simulink model "nms3D_2021"  (R2021a)
settings: Solver=ode15s  StartTime=0.0  StopTime=2  MaxStep=1e-2  RelTol=1e-2
StartFcn:
  | tic
StopFcn:
  | toc
  | 
  | 
  | %if GimbalLockFlag
  |  % fprintf(2, 'Almost reached Gimbal Lock of IMU. Simulation stopped.\n')
  | %end
  | 
  | %fprintf('Elapsed time: %4.2f sec (%4.2f%% realtime)\n', a, tout(end)/a*100)
values from neighbouring files (symbols this model uses):
  Balance02 = pMod(24:29)    [AssignSimulinkParams.m]    (also in assign_parameters.m = param(26:29))
  Balance13 = pMod(30:35)    [AssignSimulinkParams.m]    (also in assign_parameters.m = param(30:33))
  BalanceTrunk = pMod(22:23)    [AssignSimulinkParams.m]    (also in assign_parameters.m = param(22:23))
  BalanceTrunkLat = param(24:25)    [assign_parameters.m]
  BalanceTrunkLatOld = pMod(43:46)    [AssignSimulinkParams.m]    (also in assign_parameters.m = param(43:46))
  BalanceTrunkOld = param(49:53)    [assign_parameters.m]
  BasisStim = pMod(1:11)    [AssignSimulinkParams.m]    (also in assign_parameters.m = param(1:11))
  CompliantLeg = pMod(12:14)    [AssignSimulinkParams.m]    (also in assign_parameters.m = param(12:14))
  CompliantLegLat = pMod(15)    [AssignSimulinkParams.m]    (also in assign_parameters.m = param(15))
  PreventKneeOverextension = pMod(16:21)    [AssignSimulinkParams.m]    (also in assign_parameters.m = param(16:21))
  SwingCompLatOld = param(47:48)    [assign_parameters.m]
  Target02 = pMod(36:38)    [AssignSimulinkParams.m]    (also in assign_parameters.m = param(34:36))
  Target02_va = pMod(49:54)    [AssignSimulinkParams.m]    (also in assign_parameters.m = param(60:65))
  Target13 = pMod(39:41)    [AssignSimulinkParams.m]    (also in assign_parameters.m = param(37:39))
  Target13_va = pMod(55:60)    [AssignSimulinkParams.m]    (also in assign_parameters.m = param(66:71))
  theta0_world = param(59)    [assign_parameters.m]
  WramameiSL_1000 = readmatrix('WSL_1000_Norm_Sigmoid_MSE_cont.csv')    [nms3D_prep.m]
  ZramameiSL_1000 = readmatrix('ZSL_1000_Norm_Sigmoid_MSE_cont.csv')    [nms3D_prep.m]
undefined symbols (not defined in the file or in its folder): ICs, mParams, X, Y, Z
libraries: nesl_utility x106, sm_lib x87, simulink x70, eeGeneralControl x28, robotmaniplib x14, dspinverses x10, robotcorelib x5, dspmathops x3, vrlib x1, pid_lib x1
(part 7 of 8)

== system nms3D_2021/Supraspinal Level/Subsystem/Stance Leg Control/PD-Controller For Saggital Trunk Balance ==
  Gain : Gain  Gain=-1
  Low-Pass Filter (Discrete or Continuous) : eeGeneralControl/Low-Pass Filter (Discrete or Continuous)  K=1  T=0.01  B=inf  A=-inf  init_option=Inherited from block input  x0=0  Ts=-1
  Minus : Sum  Inputs=+-
  PID Controller : pid_lib/PID Controller  Controller=PD  Form=Parallel  TimeDomain=Continuous-time  UseExternalTs=off  SampleTime=-1  IntegratorMethod=Forward Euler  FilterMethod=Forward Euler  ControllerParametersSource=internal  P=40  I=0  D=80  UseFilter=on  N=100  TunerSelectOption=Transfer Function Based (PID Tuner App)  ZeroCross=off  InitialConditionSource=internal  InitialConditionForIntegrator=0  InitialConditionForFilter=0  DifferentiatorICPrevScaledInput=0  ExternalReset=none  TrackingMode=off  Kt=1  LimitOutput=off  SatLimitsSource=internal  UpperSaturationLimit=inf  LowerSaturationLimit=-inf  LinearizeAsGain=on  AntiWindupMode=none  Kb=1  POutMin=[]  POutMax=[]  IOutMin=[]  IOutMax=[]  DOutMin=[]  DOutMax=[]  NOutMin=[]  NOutMax=[]  SumOutMin=[]  SumOutMax=[]  SaturationOutMin=[]  SaturationOutMax=[]  PParamMin=[]  PParamMax=[]  IParamMin=[]  IParamMax=[]  DParamMin=[]  DParamMax=[]  NParamMin=[]  NParamMax=[]  KbParamMin=[]  KbParamMax=[]  KtParamMin=[]  KtParamMax=[]  KbOutMin=[]  KbOutMax=[]  KtOutMin=[]  KtOutMax=[]  IntegratorOutMin=[]  IntegratorOutMax=[]  FilterOutMin=[]  FilterOutMax=[]  SumI1OutMin=[]  SumI1OutMax=[]  SumI2OutMin=[]  SumI2OutMax=[]  SumI3OutMin=[]  SumI3OutMax=[]  SumI4OutMin=[]  SumI4OutMax=[]  SumDOutMin=[]  SumDOutMax=[]  DifferentiatorOutMin=[]  DifferentiatorOutMax=[]  FilterDiffOutCoefMin=[]  FilterDiffOutCoefMax=[]  ReciprocalOutMin=[]  ReciprocalOutMax=[]  SumDenOutMin=[]  SumDenOutMax=[]  SumNumOutMin=[]  SumNumOutMax=[]  DivideOutMin=[]  DivideOutMax=[]  UdiffTsProdOutMin=[]  UdiffTsProdOutMax=[]  NTsProdOutMin=[]  NTsProdOutMax=[]  UintegralTsProdOutMin=[]  UintegralTsProdOutMax=[]  UngainTsProdOutMin=[]  UngainTsProdOutMax=[]  IntegratorContinuousStateAttributes=''  IntegratorStateMustResolveToSignalObject=off  IntegratorRTWStateStorageClass=Auto  FilterContinuousStateAttributes=''  FilterStateMustResolveToSignalObject=off  FilterRTWStateStorageClass=Auto  ParallelPVariant=InternalParameters  IdealPVariant=Disabled  IVariant=Disabled  DVariant=InternalParameters  IntegratorVariant=Disabled  SatVariant=Disabled  AWVariant=Disabled  PCopyVariant=Disabled  TRVariant=Disabled  FdbkBlocksVariant=Forward  IdealPFdbkVariant=Disabled  SatFdbkVariant=Disabled  DerivativeFilterVariant=ContFilter  NVariant=InternalParameters  NCopyVariant=Disabled  FilterICVariant=InternalICsFilter  IntegratorICVariant=Disabled  ExternalResetVariant=Disabled  TRSumVariant=Passthrough  SumFdbkVariant=Disabled  SumVariant=Sum_PD  TsampFilterVariant=InternalTs  TsampNgainVariant=Passthrough  TsampIntegralVariant=Disabled_SignalSpec  ExternalSaturationOutDataTypeStr=Inherit: Same as second input
  Scope{,1..3} (4 alike) : Scope
  To Workspace6 : ToWorkspace  VariableName=RotSag  SampleTime=-1
      settings: Save2DSignal=2-D array (concatenate along first dimension)
  PD Input : Outport
  wires:
  Gain/1 -> Low-Pass Filter (Discrete or Continuous)/1
  Minus/1 -> Scope2/1, PID Controller/1
  [TrunkRot_sag] -> To Workspace6/1, Minus/1, Scope/1
  PID Controller/1 -> Scope3/1, Gain/1
  [theta0_world] -> Scope1/1, Minus/2
  Low-Pass Filter (Discrete or Continuous)/1 -> PD Input/1

== system nms3D_2021/Supraspinal Level/Subsystem/Stance Leg Control/Stance Leg ==
  left/right : Inport
  Balance Control [Ankle Strategy] : Inport  Port=2
  PD Input : Inport  Port=3
  Foot Orientation Left : Subsystem
  Foot Orientation Right : Subsystem
  Inverse Dynamics Left Leg : Subsystem
  Mux : Mux  Inputs=2
  Mux1 : Mux  Inputs=2
  NOT : Logic  Operator=NOT  AllPortsSameDT=off  OutDataTypeStr=boolean
  NOT2 : Logic  Operator=NOT  AllPortsSameDT=off  OutDataTypeStr=boolean
  Selector : Selector  InputPortWidth=5  IndexOptions=Index vector (dialog)  Indices=[5 4 3 2 1]  OutputSizes=1
  Selector1 : Selector  InputPortWidth=5  IndexOptions=Index vector (dialog)  Indices=[5 4 3 2 1]  OutputSizes=1
  Subsystem : Subsystem
  Transpose : Math  Operator=transpose  SaturateOnIntegerOverflow=on
  long delay 1 : eeGeneralControl/Low-Pass Filter (Discrete or Continuous)  K=1  T=mParams.control.delays.long  B=inf  A=-inf  init_option=Inherited from block input  x0=0  Ts=0
  long delay 2 : eeGeneralControl/Low-Pass Filter (Discrete or Continuous)  K=1  T=mParams.control.delays.long  B=inf  A=-inf  init_option=Inherited from block input  x0=0  Ts=0
  long delay 4 : eeGeneralControl/Low-Pass Filter (Discrete or Continuous)  K=1  T=mParams.control.delays.long  B=inf  A=-inf  init_option=Inherited from block input  x0=0  Ts=0
  Stance Torques Left : Outport
  Stance Torques Right : Outport  Port=2
  wires:
  Selector/1 -> Mux/2
  Selector1/1 -> Mux1/2
  [R_body] -> long delay 4/1
  left/right/1 -> NOT/1, NOT2/1, Inverse Dynamics Left Leg/2(left/right)
  Transpose/1 -> Foot Orientation Right/1(R Pelvis), Foot Orientation Left/1(R Pelvis)
  Foot Orientation Left/1(Orientation Foot (Z)) -> Mux1/1
  Foot Orientation Right/1(Foot Orientation (Z)) -> Mux/1
  Balance Control [Ankle Strategy]/1 -> Inverse Dynamics Left Leg/3(Task), Subsystem/4(Task)
  Inverse Dynamics Left Leg/1(Stance Torques Left) -> Stance Torques Left/1
  Mux/1 -> Subsystem/1(Config [5])
  NOT2/1 -> Subsystem/3(left/right)
  Subsystem/1(Stance Torques Right) -> Stance Torques Right/1
  Mux1/1 -> Inverse Dynamics Left Leg/1(Config [5])
  long delay 1/1 -> Selector1/1
  long delay 2/1 -> Selector/1
  long delay 4/1 -> Transpose/1
  [Llegq] -> long delay 1/1
  [Rlegq] -> long delay 2/1
  PD Input/1 -> Subsystem/2(PD Input), Inverse Dynamics Left Leg/4(PD Input)

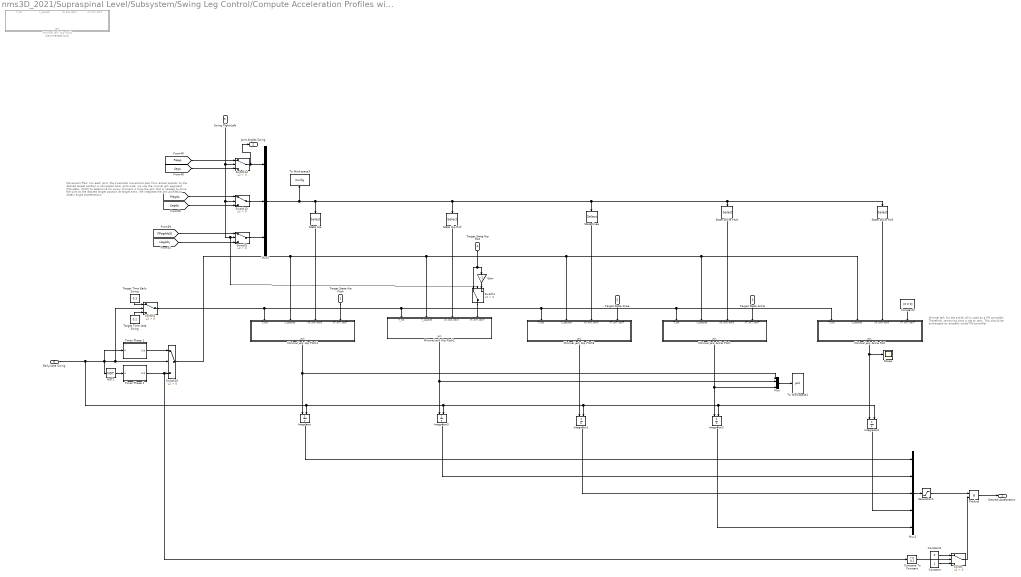
== system nms3D_2021/Supraspinal Level/Subsystem/Swing Leg Control/Compute Acceleration Profiles with Minimal Jerk Approach ==
  note: Movement Plan: For each joint, the kinematic movement plan from actual position to the desired target position is computed here. Joint-wise, we use the mininal jerk approach [Movellan, 2012] to determine for every moment in time the jerk that is needed to drive the joint to the desired target position at target time. We integrate the jerk profiles to obtain angle accelerations.
  note: Minimal Jerk for the ankle roll is used as a PD controller. Therefore, remaining time is set to zero. This should be exchanged by properly tuned PD-controller
  Target State Hip Pitch : Inport
  Target State Knee : Inport  Port=2
  Target State Ankle : Inport  Port=3
  Target State Hip Roll : Inport  Port=4
  Swing Right/Left : Inport  Port=5
  Early/Late Swing : Inport  Port=6
  " Timer Phase 1" : Subsystem
  " Timer Phase 2" : Subsystem
  Compare To Constant : simulink/Logic and Bit Operations/Compare To Constant  relop=>=  const=0.2  OutDataTypeStr=boolean  ZeroCross=off
  Constant : Constant
  Constant1 : Constant  Value=0
  Constant2 : Constant  Value=[0 0 0]
  Gain : Gain  Gain=-1
  Integrator{,1..4} (5 alike) : Integrator  ExternalReset=either  ZeroCross=off
  Minimal jerk Ankle Pitch : Subsystem
  Minimal jerk Ankle Roll : Subsystem
  Minimal jerk Hip Pitch1 : Subsystem
  Minimal jerk Hip Pitch2 : Subsystem
  Minimal jerk Hip Pitch3 : Subsystem
  Minimal jerk Hip Roll4 : Subsystem  Commented=on
  Mux : Mux
  Mux1 : Mux  Inputs=5
  Mux5 : Mux  Inputs=3
  NOT1 : Logic  Operator=NOT  AllPortsSameDT=off  OutDataTypeStr=boolean
  Product : Product
  Saturation1 : Saturate  UpperLimit=2000  LowerLimit=-2000  ZeroCross=off
  Scope : Scope
  State Ankle Pitch : Selector  InputPortWidth=15  IndexOptions=Index vector (dialog)  Indices=[5 10 15]  OutputSizes=1
  State Ankle Roll : Selector  InputPortWidth=15  IndexOptions=Index vector (dialog)  Indices=[4 9 14]  OutputSizes=1
  State Hip : Selector  InputPortWidth=15  IndexOptions=Index vector (dialog)  Indices=[1 6 11]  OutputSizes=1
  State Hip Roll : Selector  InputPortWidth=15  IndexOptions=Index vector (dialog)  Indices=[2 7 12 ]  OutputSizes=1
  State Knee : Selector  InputPortWidth=15  IndexOptions=Index vector (dialog)  Indices=[3 8 13 ]  OutputSizes=1
  Switch{,1..2,5,13..14,16} (7 alike) : Switch  Criteria=u2 > Threshold
  Target Time Early Swing : Constant  Value=0.3
  Target Time Late Swing : Constant  Value=0.2
  To Workspace1 : ToWorkspace  VariableName=Jerk  SampleTime=-1
      settings: Save2DSignal=2-D array (concatenate along first dimension)
  To Workspace3 : ToWorkspace  VariableName=Config  SampleTime=-1
      settings: Save2DSignal=2-D array (concatenate along first dimension)
  "Desired Acceleration " : Outport
  Joint Angles Swing : Outport  Port=2
  wires:
  State Hip/1 -> Minimal jerk Hip Pitch1/3("x0, dx0, ddx0")
  NOT1/1 -> " Timer Phase 2"/1(R)
  Mux1/1 -> Saturation1/1
  Switch2/1 -> Minimal jerk Hip Pitch1/1(T_tot), Minimal jerk Hip Pitch2/1(T_tot), Minimal jerk Ankle Roll/1(T_tot), Minimal jerk Ankle Pitch/1(T_tot), Minimal jerk Hip Pitch3/1(T_tot)
  Target State Hip Pitch/1 -> Minimal jerk Hip Pitch1/4("xT, dxT, ddxT")
  Target State Knee/1 -> Minimal jerk Hip Pitch3/4("xT, dxT, ddxT")
  Integrator1/1 -> Mux1/3
  Switch5/1 -> Mux5/3
  State Knee/1 -> Minimal jerk Hip Pitch3/3("x0, dx0, ddx0")
  Target State Ankle/1 -> Minimal jerk Ankle Pitch/4("xT, dxT, ddxT")
  Integrator/1 -> Mux1/1
  Switch14/1 -> Joint Angles Swing/1, Mux5/1
  Integrator2/1 -> Mux1/5
  State Ankle Pitch/1 -> Minimal jerk Ankle Pitch/3("x0, dx0, ddx0")
  Switch13/1 -> Mux5/2
  Early/Late Swing/1 -> Switch2/2, Switch16/2, NOT1/1, " Timer Phase 1"/1(R), Integrator3/2, Integrator2/2, Integrator4/2, Integrator1/2, Integrator/2
  Swing Right/Left/1 -> Switch14/2, Switch13/2, Switch1/2, Switch5/2
  Switch16/1 -> Minimal jerk Hip Pitch1/2(t_passed), Minimal jerk Hip Pitch2/2(t_passed), Minimal jerk Ankle Pitch/2(t_passed), Minimal jerk Ankle Roll/2(t_passed), Minimal jerk Hip Pitch3/2(t_passed)
  State Hip Roll/1 -> Minimal jerk Hip Pitch2/3("x0, dx0, ddx0")
  Integrator3/1 -> Mux1/2
  Switch1/1 -> Minimal jerk Hip Pitch2/4("xT, dxT, ddxT")
  Target State Hip Roll/1 -> Gain/1, Switch1/1
  Gain/1 -> Switch1/3
  Target Time Early Swing/1 -> Switch2/1
  Target Time Late Swing/1 -> Switch2/3
  " Timer Phase 1"/1(Out) -> Switch16/1
  " Timer Phase 2"/1(Out) -> Compare To Constant/1, Switch16/3
  Mux5/1 -> State Hip Roll/1, State Ankle Roll/1, State Ankle Pitch/1, State Knee/1, State Hip/1, To Workspace3/1
  Mux/1 -> To Workspace1/1
  Minimal jerk Hip Pitch1/1(jerk) -> Mux/1, Integrator/1
  Minimal jerk Hip Pitch2/1(jerk) -> Mux/2, Integrator3/1
  Minimal jerk Hip Pitch3/1(jerk) -> Integrator1/1
  Minimal jerk Ankle Pitch/1(jerk) -> Mux/4, Integrator2/1
  Saturation1/1 -> Product/1
  Compare To Constant/1 -> Switch/2
  Constant/1 -> Switch/3
  Constant1/1 -> Switch/1
  Switch/1 -> Product/2
  Product/1 -> "Desired Acceleration "/1
  [Rlegq] -> Switch14/1
  [Llegq] -> Switch14/3
  [Rlegdq] -> Switch13/1
  [Llegdq] -> Switch13/3
  [Rlegddq5] -> Switch5/1
  [Llegddq] -> Switch5/3
  Constant2/1 -> Minimal jerk Ankle Roll/4("xT, dxT, ddxT")
  State Ankle Roll/1 -> Minimal jerk Ankle Roll/3("x0, dx0, ddx0")
  Minimal jerk Ankle Roll/1(jerk) -> Scope/1, Integrator4/1
  Integrator4/1 -> Mux1/4

== system nms3D_2021/Supraspinal Level/Subsystem/Swing Leg Control/Compute Target States ==
  note: Target Joint States: Target joint angles, angle velocities and angle acceleration are defined here. For knee and ankle, values are constant. For hip pitch and hip roll, values are computed using the Balance Control mechanism from [Yin et. al. 2007].
      | Low pass filters are added here to compensate for abrupt changes in target angles at transitions between early and late swing.
  Left/Right : Inport
  Early/Late : Inport  Port=2
  Balance Control lateral : Subsystem
  Balance Control saggital : Subsystem
  Constant13 : Constant  Value=pi
  Gain3 : Gain  Gain=-1
  Low-Pass Filter (Discrete or Continuous)1 : eeGeneralControl/Low-Pass Filter (Discrete or Continuous)  K=1  T=0.1  B=inf  A=-inf  init_option=Inherited from block input  x0=-13  Ts=0
  Low-Pass Filter (Discrete or Continuous)2 : eeGeneralControl/Low-Pass Filter (Discrete or Continuous)  K=1  T=0.1  B=inf  A=-inf  init_option=Inherited from block input  x0=-13  Ts=0
  Minus1 : Sum
  Minus8 : Sum  Inputs=+++
  Mux{2..3,5..6} (4 alike) : Mux  Inputs=3
  Product : Product
  Sign : Signum  ZeroCross=off
  Hip Pitch Target : Outport
  Knee Target : Outport  Port=2
  Ankle Target : Outport  Port=3
  Hip Roll Target : Outport  Port=4
  wires:
  [TrunkRot_sag] -> Minus8/3
  Left/Right/1 -> Balance Control lateral/1(Left/Right), Balance Control saggital/1(Left/Right)
  Gain3/1 -> Minus8/1
  [swk] -> Mux5/1
  Balance Control lateral/1(theta_Hip_swing_target) -> Sign/1, Minus1/1
  Balance Control saggital/1(theta_Hip_swing_target) -> Gain3/1
  Mux5/1 -> Knee Target/1
  Constant13/1 -> Minus8/2
  [TrunkRot_lat] -> Minus1/2
  Mux2/1 -> Low-Pass Filter (Discrete or Continuous)2/1
  Mux6/1 -> Ankle Target/1
  Minus1/1 -> Mux2/1
  Low-Pass Filter (Discrete or Continuous)2/1 -> Hip Roll Target/1
  [swk_v] -> Mux5/2
  [swk_a] -> Mux5/3
  [swa] -> Mux6/1
  [swa_v] -> Mux6/2
  [swa_a] -> Mux6/3
  [swh_lat_a] -> Mux2/3
  [swh_lat_v] -> Product/1
  Product/1 -> Mux2/2
  Sign/1 -> Product/2
  Minus8/1 -> Mux3/1
  [swh_v] -> Mux3/2
  [swh_a] -> Mux3/3
  Mux3/1 -> Low-Pass Filter (Discrete or Continuous)1/1
  Low-Pass Filter (Discrete or Continuous)1/1 -> Hip Pitch Target/1
  Early/Late/1 -> Balance Control saggital/2(Early Late)

== system nms3D_2021/Supraspinal Level/Subsystem/Swing Leg Control/Inverse Dynamics: Left Leg ==
  Desired Acceleration : Inport
  Enable : Inport  Port=2
  Inverse Dynamics : Subsystem
  Sensor Data from Body Layer : Subsystem
  Desired Torques : Outport
  Interaction Wrench : Outport  Port=2
  wires:
  Inverse Dynamics/1(" Desired Torques") -> Desired Torques/1
  Desired Acceleration/1 -> Inverse Dynamics/8(Desired Acceleration [rad/s^2])
  Sensor Data from Body Layer/4(" Rotation Trunk [rad]") -> Inverse Dynamics/4(Rotation Trunk [rad])
  Sensor Data from Body Layer/2(Joint Angle Velocities [rad/s]) -> Inverse Dynamics/2(Joint Angle Velocities [rad/s])
  Sensor Data from Body Layer/1(Joint Angles [rad]) -> Inverse Dynamics/1(Joint Angles [rad])
  Sensor Data from Body Layer/6(Rotation Velocity Trunk [rad/s]) -> Inverse Dynamics/6(Rotation Velocity Trunk [rad/s])
  Sensor Data from Body Layer/5(Trunk Position [m]) -> Inverse Dynamics/5(Trunk Position [m])
  Sensor Data from Body Layer/7(Trunk Velocity [m/s]) -> Inverse Dynamics/7(Trunk Velocity [m/s])
  Enable/1 -> Inverse Dynamics/Enable
  Inverse Dynamics/2(Interaction Wrench) -> Interaction Wrench/1
  Sensor Data from Body Layer/3(Joint Angle Accelerations [rad/s^2]) -> Inverse Dynamics/3(Joint  Acceleration [rad/s^2])

== system nms3D_2021/Supraspinal Level/Subsystem/Swing Leg Control/Inverse Dynamics: Right Leg ==
  Desired Acceleration : Inport
  Enable : Inport  Port=2
  Inverse Dynamics1 : Subsystem
  Sensor Data from Body Layer1 : Subsystem
  Desired Torques : Outport
  Interaction Wrench : Outport  Port=2
  wires:
  Inverse Dynamics1/1(" Desired Torques") -> Desired Torques/1
  Enable/1 -> Inverse Dynamics1/Enable
  Inverse Dynamics1/2(Interaction Wrench) -> Interaction Wrench/1
  Sensor Data from Body Layer1/1(Joint Angles [rad]) -> Inverse Dynamics1/1(Joint Angles [rad])
  Sensor Data from Body Layer1/2(Joint Angle Velocities [rad/s]) -> Inverse Dynamics1/2(Joint Angle Velocities [rad/s])
  Sensor Data from Body Layer1/3(Joint Angle Accelerations [rad/s^2]) -> Inverse Dynamics1/3(Joint  Acceleration [rad/s^2])
  Sensor Data from Body Layer1/4(" Rotation Trunk [rad]") -> Inverse Dynamics1/4(Rotation Trunk [rad])
  Sensor Data from Body Layer1/5(Trunk Position [m]) -> Inverse Dynamics1/5(Trunk Position [m])
  Sensor Data from Body Layer1/6(Rotation Velocity Trunk [rad/s]) -> Inverse Dynamics1/6(Rotation Velocity Trunk [rad/s])
  Sensor Data from Body Layer1/7(Trunk Velocity [m/s]) -> Inverse Dynamics1/7(Trunk Velocity [m/s])
  Desired Acceleration/1 -> Inverse Dynamics1/8(Desired Acceleration [rad/s^2])

== system nms3D_2021/Supraspinal Level/Subsystem/Compute positives forces that generate desired torque profiles1/Left/sigmoid ==
  In1 : Inport
  Add : Sum
  Constant : Constant
  Constant1 : Constant
  Divide : Product  Inputs=*/
  Exp : Math  SaturateOnIntegerOverflow=on
  Gain : Gain  Gain=-1
  Out1 : Outport
  wires:
  Constant/1 -> Divide/1
  Constant1/1 -> Add/1
  In1/1 -> Gain/1
  Gain/1 -> Exp/1
  Exp/1 -> Add/2
  Add/1 -> Divide/2
  Divide/1 -> Out1/1

== system nms3D_2021/Supraspinal Level/Subsystem/Compute positives forces that generate desired torque profiles1/Right/sigmoid ==
  In1 : Inport
  Add : Sum
  Constant : Constant
  Constant1 : Constant
  Divide : Product  Inputs=*/
  Exp : Math  SaturateOnIntegerOverflow=on
  Gain : Gain  Gain=-1
  Out1 : Outport
  wires:
  Constant/1 -> Divide/1
  Constant1/1 -> Add/1
  In1/1 -> Gain/1
  Gain/1 -> Exp/1
  Exp/1 -> Add/2
  Add/1 -> Divide/2
  Divide/1 -> Out1/1

== system nms3D_2021/Supraspinal Level/Subsystem/Stance Leg Control/Balance Control Equation [Ankle Strategy]/mean (1s) ==
  u : Inport
  Constant : Constant  Value=101
  Divide2 : Product  Inputs=*/
  Scope1 : Scope
  Sum of Elements : Sum  Inputs=+  CollapseMode=Specified dimension  AccumDataTypeStr=double
  Tapped Delay : simulink/Discrete/Tapped Delay  vinit=1.3  samptime=0.01  NumDelays=100  DelayOrder=Newest  includeCurrent=off
  Vector Concatenate : Concatenate
  u_average : Outport
  wires:
  Tapped Delay/1 -> Vector Concatenate/2
  Vector Concatenate/1 -> Sum of Elements/1
  Sum of Elements/1 -> Divide2/1
  Divide2/1 -> Scope1/1, u_average/1
  u/1 -> Tapped Delay/1, Vector Concatenate/1
  Constant/1 -> Divide2/2

== system nms3D_2021/Supraspinal Level/Subsystem/Stance Leg Control/Coordiante Transform Interaction Wrenches/Create Adjoint ==
  R : Inport
  Constant3 : Constant  Value=zeros(3,3)
  Matrix Concatenate : Concatenate  Mode=Multidimensional array  ConcatenateDimension=2
  Matrix Concatenate1 : Concatenate  Mode=Multidimensional array  ConcatenateDimension=2
  Matrix Concatenate2 : Concatenate  Mode=Multidimensional array
  Ad(R) : Outport
  wires:
  Matrix Concatenate2/1 -> Ad(R)/1
  Matrix Concatenate1/1 -> Matrix Concatenate2/2
  Constant3/1 -> Matrix Concatenate1/1, Matrix Concatenate/2
  Matrix Concatenate/1 -> Matrix Concatenate2/1
  R/1 -> Matrix Concatenate1/2, Matrix Concatenate/1

== system nms3D_2021/Supraspinal Level/Subsystem/Stance Leg Control/Coordiante Transform Interaction Wrenches/Transform  Velocity from world to body  ==
  body-world jacobian : Inport
  translational velocity [world] : Inport  Port=2
  rotational velocity [world] : Inport  Port=3
  Matrix Multiply1 : Product  Multiplication=Matrix(*)
  Mux6 : Mux  Inputs=2
  Pseudoinverse1 : dspinverses/Pseudoinverse  wanterr=off  SimulateUsing=Interpreted execution
      settings: SourceProductBaseCode=DS
  select Rotation : Selector  InputPortWidth=6  IndexOptions=Index vector (dialog)  Indices=[4 5 6]  OutputSizes=1
  select Translation : Selector  InputPortWidth=6  IndexOptions=Index vector (dialog)  Indices=[1 2 3]  OutputSizes=1
  Translational Velocity [body] : Outport
  Rotational Velocity [body] : Outport  Port=2
  wires:
  translational velocity [world]/1 -> Mux6/2
  body-world jacobian/1 -> Pseudoinverse1/1
  Mux6/1 -> Matrix Multiply1/2
  rotational velocity [world]/1 -> Mux6/1
  Pseudoinverse1/1 -> Matrix Multiply1/1
  Matrix Multiply1/1 -> select Rotation/1, select Translation/1
  select Rotation/1 -> Rotational Velocity [body]/1
  select Translation/1 -> Translational Velocity [body]/1

== system nms3D_2021/Supraspinal Level/Subsystem/Stance Leg Control/Coordiante Transform Interaction Wrenches/transform wrench from body to world frame1 ==
  "CoM Pos " : Inport
  CoM Rot : Inport  Port=2
  wrench [rbt model] : Inport  Port=3
  Get Jacobian : robotmaniplib/Get Jacobian  RigidBodyTree=model_trunk  EndEffector=Trunk  SimulateUsing=Code generation
      settings: SourceProductBaseCode=RO
  Matrix Multiply : Product  Multiplication=Matrix(*)
  Mux5 : Mux  Inputs=2
  Pseudoinverse : dspinverses/Pseudoinverse  wanterr=off  SimulateUsing=Interpreted execution
      settings: SourceProductBaseCode=DS
  Transpose : Math  Operator=transpose  SaturateOnIntegerOverflow=on
  select forces : Selector  InputPortWidth=6  IndexOptions=Index vector (dialog)  Indices=[4 5 6]  OutputSizes=1
  select torques : Selector  InputPortWidth=6  IndexOptions=Index vector (dialog)  Indices=[1 2 3]  OutputSizes=1
  body-world jacobian : Outport
  torque : Outport  Port=2
  force : Outport  Port=3
  wires:
  CoM Rot/1 -> Mux5/2
  wrench [rbt model]/1 -> Matrix Multiply/2
  "CoM Pos "/1 -> Mux5/1
  Transpose/1 -> Pseudoinverse/1
  select forces/1 -> force/1
  select torques/1 -> torque/1
  Get Jacobian/1 -> body-world jacobian/1, Transpose/1
  Mux5/1 -> Get Jacobian/1
  Matrix Multiply/1 -> select torques/1, select forces/1
  Pseudoinverse/1 -> Matrix Multiply/1

== system nms3D_2021/Supraspinal Level/Subsystem/Stance Leg Control/Stance Leg/Foot Orientation Left ==
  R Pelvis : Inport
  Coordinate Transformation Conversion1 : robotcorelib/Coordinate Transformation Conversion  InputRepresentation=Rotation Matrix  InputEulerSequence=ZYX  ShowTrVecInputPort=on  OutputRepresentation=Euler Angles  OutputEulerSequence=XYZ  ShowTrVecOutputPort=on  SimulateUsing=Code generation
      settings: SourceProductBaseCode=NV,RO,RR,UV
  Matrix Multiply : Product  Multiplication=Matrix(*)
  Selector2 : Selector  InputPortWidth=3  IndexOptions=Index vector (dialog)  Indices=[ 3]  OutputSizes=1
  Orientation Foot (Z) : Outport
  wires:
  Coordinate Transformation Conversion1/1 -> Selector2/1
  Matrix Multiply/1 -> Coordinate Transformation Conversion1/1
  Selector2/1 -> Orientation Foot (Z)/1
  R Pelvis/1 -> Matrix Multiply/1
  [RotationMatrixLeftFoot] -> Matrix Multiply/2

== system nms3D_2021/Supraspinal Level/Subsystem/Stance Leg Control/Stance Leg/Foot Orientation Right ==
  R Pelvis : Inport
  Coordinate Transformation Conversion3 : robotcorelib/Coordinate Transformation Conversion  InputRepresentation=Rotation Matrix  InputEulerSequence=ZYX  ShowTrVecInputPort=on  OutputRepresentation=Euler Angles  OutputEulerSequence=XYZ  ShowTrVecOutputPort=on  SimulateUsing=Code generation
      settings: SourceProductBaseCode=NV,RO,RR,UV
  Matrix Multiply1 : Product  Multiplication=Matrix(*)
  Selector3 : Selector  InputPortWidth=3  IndexOptions=Index vector (dialog)  Indices=[ 3]  OutputSizes=1
  Foot Orientation (Z) : Outport
  wires:
  R Pelvis/1 -> Matrix Multiply1/1
  Selector3/1 -> Foot Orientation (Z)/1
  Coordinate Transformation Conversion3/1 -> Selector3/1
  [RotationMatrixRightFoot] -> Matrix Multiply1/2
  Matrix Multiply1/1 -> Coordinate Transformation Conversion3/1

== system nms3D_2021/Supraspinal Level/Subsystem/Stance Leg Control/Stance Leg/Inverse Dynamics Left Leg ==
  Config [5] : Inport
  left/right : Inport  Port=2
  Task : Inport  Port=3
  PD Input : Inport  Port=4
  Left Leg Ball : Subsystem
  Low-Pass Filter (Discrete or Continuous) : eeGeneralControl/Low-Pass Filter (Discrete or Continuous)  K=1  T=0.01  B=150  A=-150  init_option=Inherited from block input  x0=0  Ts=0
  Product : Product
  Selector4 : Selector  InputPortWidth=6  IndexOptions=Index vector (dialog)  Indices=[6 5 4 3 2]  OutputSizes=1
  Stance Torques Left : Outport
  wires:
  Product/1 -> Selector4/1
  Selector4/1 -> Low-Pass Filter (Discrete or Continuous)/1
  Left Leg Ball/1(Push-Off Left (Ball)) -> Product/1
  left/right/1 -> Product/2, Left Leg Ball/Enable
  Config [5]/1 -> Left Leg Ball/1(Config)
  Task/1 -> Left Leg Ball/2(Task)
  Low-Pass Filter (Discrete or Continuous)/1 -> Stance Torques Left/1
  PD Input/1 -> Left Leg Ball/3(PD Input)

== system nms3D_2021/Supraspinal Level/Subsystem/Stance Leg Control/Stance Leg/Subsystem ==
  Config [5] : Inport
  PD Input : Inport  Port=2
  left/right : Inport  Port=3
  Task : Inport  Port=4
  Low-Pass Filter (Discrete or Continuous)1 : eeGeneralControl/Low-Pass Filter (Discrete or Continuous)  K=1  T=0.01  B=150  A=-150  init_option=Inherited from block input  x0=0  Ts=0
  Product1 : Product
  Right Leg Ball : Subsystem
  Selector : Selector  InputPortWidth=6  IndexOptions=Index vector (dialog)  Indices=[2 3 4 5 6]  OutputSizes=1
  Selector5 : Selector  InputPortWidth=6  IndexOptions=Index vector (dialog)  Indices=[6 5 4 3 2]  OutputSizes=1
  Stance Torques Right : Outport
  wires:
  Selector5/1 -> Low-Pass Filter (Discrete or Continuous)1/1
  Low-Pass Filter (Discrete or Continuous)1/1 -> Stance Torques Right/1
  left/right/1 -> Product1/2, Right Leg Ball/Enable
  Task/1 -> Right Leg Ball/2(Task)
  Right Leg Ball/1(Push-Off Right (Ball)) -> Product1/1
  Product1/1 -> Selector5/1
  Config [5]/1 -> Right Leg Ball/1(Config)
  PD Input/1 -> Right Leg Ball/3(PD Input)

== system nms3D_2021/Supraspinal Level/Subsystem/Swing Leg Control/Compute Acceleration Profiles with Minimal Jerk Approach/ Timer Phase 1 ==
  R : Inport
  Clock1 : Clock
  Clock3 : Clock
      settings: Decimation=4
  NOT : Logic  Operator=NOT  AllPortsSameDT=off  OutDataTypeStr=boolean
  Resettable Subsystem : Subsystem  TreatAsAtomicUnit=on
  Sum1 : Sum  Inputs=|+-  InputSameDT=on  SaturateOnIntegerOverflow=on  OutDataTypeStr=Inherit: Same as first input
  Switch2 : Switch  Criteria=u2 > Threshold  RndMeth=Zero
  Out : Outport  VectorParamsAs1DForOutWhenUnconnected=off
  wires:
  Clock1/1 -> Sum1/1
  Clock3/1 -> Switch2/3, Resettable Subsystem/1(In1)
  Sum1/1 -> Out/1
  R/1 -> NOT/1, Switch2/2
  Switch2/1 -> Sum1/2
  Resettable Subsystem/1(Out1) -> Switch2/1
  NOT/1 -> Resettable Subsystem/Enable

== system nms3D_2021/Supraspinal Level/Subsystem/Swing Leg Control/Compute Acceleration Profiles with Minimal Jerk Approach/ Timer Phase 2 ==
  R : Inport
  Clock1 : Clock
  Clock3 : Clock
      settings: Decimation=4
  NOT : Logic  Operator=NOT  AllPortsSameDT=off  OutDataTypeStr=boolean
  Resettable Subsystem : Subsystem  TreatAsAtomicUnit=on
  Sum1 : Sum  Inputs=|+-  InputSameDT=on  SaturateOnIntegerOverflow=on  OutDataTypeStr=Inherit: Same as first input
  Switch2 : Switch  Criteria=u2 > Threshold  RndMeth=Zero
  Out : Outport  VectorParamsAs1DForOutWhenUnconnected=off
  wires:
  Clock1/1 -> Sum1/1
  Clock3/1 -> Switch2/3, Resettable Subsystem/1(In1)
  Sum1/1 -> Out/1
  R/1 -> NOT/1, Switch2/2
  Switch2/1 -> Sum1/2
  Resettable Subsystem/1(Out1) -> Switch2/1
  NOT/1 -> Resettable Subsystem/Enable

== system nms3D_2021/Supraspinal Level/Subsystem/Swing Leg Control/Compute Acceleration Profiles with Minimal Jerk Approach/Minimal jerk Ankle Pitch ==
  T_tot : Inport
  t_passed : Inport  Port=2
  "x0, dx0, ddx0" : Inport  Port=3
  "xT, dxT, ddxT" : Inport  Port=4
  Compare To Constant : simulink/Logic and Bit Operations/Compare To Constant  relop=>=  const=mParams.control.timelimit  OutDataTypeStr=boolean
  Constant : Constant  Value=mParams.control.timelimit
  Constant1 : Constant  Value=0
  Demux : Demux  Outputs=3
  Demux1 : Demux  Outputs=3
  Enabled Subsystem : Subsystem  TreatAsAtomicUnit=on
  Minimal Jerk : Subsystem
  Minimal Jerk Parameters [Movellan] : Subsystem
  Minus : Sum  Inputs=+-
  Minus1 : Sum  Inputs=+-
  Switch : Switch
  jerk : Outport
  wires:
  Minimal Jerk/1(j(t)) -> jerk/1
  T_tot/1 -> Minus/1
  t_passed/1 -> Minus/2
  Constant1/1 -> Switch/1
  Demux/1 -> Minimal Jerk Parameters [Movellan]/1(x0)
  Demux/2 -> Minimal Jerk Parameters [Movellan]/2(dx0)
  Demux/3 -> Minimal Jerk Parameters [Movellan]/3(ddx0)
  Demux1/1 -> Minimal Jerk Parameters [Movellan]/4(xT)
  "x0, dx0, ddx0"/1 -> Demux/1
  Demux1/2 -> Minimal Jerk Parameters [Movellan]/5(dxT)
  "xT, dxT, ddxT"/1 -> Demux1/1
  Demux1/3 -> Minimal Jerk Parameters [Movellan]/6(ddxT)
  Minimal Jerk Parameters [Movellan]/1(a) -> Enabled Subsystem/1(In1)
  Minus/1 -> Compare To Constant/1, Minus1/2, Minimal Jerk Parameters [Movellan]/7(T)
  Enabled Subsystem/1(Out1) -> Minimal Jerk/2(a [6x1])
  Compare To Constant/1 -> Switch/2, Enabled Subsystem/Enable
  Constant/1 -> Minus1/1
  Minus1/1 -> Switch/3
  Switch/1 -> Minimal Jerk/1(t)

== system nms3D_2021/Supraspinal Level/Subsystem/Swing Leg Control/Compute Acceleration Profiles with Minimal Jerk Approach/Minimal jerk Ankle Roll ==
  T_tot : Inport
  t_passed : Inport  Port=2
  "x0, dx0, ddx0" : Inport  Port=3
  "xT, dxT, ddxT" : Inport  Port=4
  Compare To Constant : simulink/Logic and Bit Operations/Compare To Constant  relop=>=  const=mParams.control.timelimit  OutDataTypeStr=boolean
  Constant : Constant  Value=mParams.control.timelimit
  Constant1 : Constant  Value=0
  Demux : Demux  Outputs=3
  Demux1 : Demux  Outputs=3
  Enabled Subsystem : Subsystem  TreatAsAtomicUnit=on
  Minimal Jerk : Subsystem
  Minimal Jerk Parameters [Movellan] : Subsystem
  Minus : Sum  Inputs=+-
  Minus1 : Sum  Inputs=+-
  Switch : Switch
  jerk : Outport
  wires:
  Minimal Jerk/1(j(t)) -> jerk/1
  T_tot/1 -> Minus/1
  t_passed/1 -> Minus/2
  Constant1/1 -> Switch/1
  Demux/1 -> Minimal Jerk Parameters [Movellan]/1(x0)
  Demux/2 -> Minimal Jerk Parameters [Movellan]/2(dx0)
  Demux/3 -> Minimal Jerk Parameters [Movellan]/3(ddx0)
  Demux1/1 -> Minimal Jerk Parameters [Movellan]/4(xT)
  "x0, dx0, ddx0"/1 -> Demux/1
  Demux1/2 -> Minimal Jerk Parameters [Movellan]/5(dxT)
  "xT, dxT, ddxT"/1 -> Demux1/1
  Demux1/3 -> Minimal Jerk Parameters [Movellan]/6(ddxT)
  Minimal Jerk Parameters [Movellan]/1(a) -> Enabled Subsystem/1(In1)
  Minus/1 -> Compare To Constant/1, Minus1/2, Minimal Jerk Parameters [Movellan]/7(T)
  Enabled Subsystem/1(Out1) -> Minimal Jerk/2(a [6x1])
  Compare To Constant/1 -> Switch/2, Enabled Subsystem/Enable
  Constant/1 -> Minus1/1
  Minus1/1 -> Switch/3
  Switch/1 -> Minimal Jerk/1(t)

== system nms3D_2021/Supraspinal Level/Subsystem/Swing Leg Control/Compute Acceleration Profiles with Minimal Jerk Approach/Minimal jerk Hip Pitch1 ==
  T_tot : Inport
  t_passed : Inport  Port=2
  "x0, dx0, ddx0" : Inport  Port=3
  "xT, dxT, ddxT" : Inport  Port=4
  Compare To Constant : simulink/Logic and Bit Operations/Compare To Constant  relop=>=  const=mParams.control.timelimit  OutDataTypeStr=boolean
  Constant : Constant  Value=mParams.control.timelimit
  Constant1 : Constant  Value=0
  Demux : Demux  Outputs=3
  Demux1 : Demux  Outputs=3
  Enabled Subsystem : Subsystem  TreatAsAtomicUnit=on
  Minimal Jerk : Subsystem
  Minimal Jerk Parameters [Movellan] : Subsystem
  Minus : Sum  Inputs=+-
  Minus1 : Sum  Inputs=+-
  Switch : Switch
  jerk : Outport
  wires:
  Minimal Jerk/1(j(t)) -> jerk/1
  T_tot/1 -> Minus/1
  t_passed/1 -> Minus/2
  Constant1/1 -> Switch/1
  Demux/1 -> Minimal Jerk Parameters [Movellan]/1(x0)
  Demux/2 -> Minimal Jerk Parameters [Movellan]/2(dx0)
  Demux/3 -> Minimal Jerk Parameters [Movellan]/3(ddx0)
  Demux1/1 -> Minimal Jerk Parameters [Movellan]/4(xT)
  "x0, dx0, ddx0"/1 -> Demux/1
  Demux1/2 -> Minimal Jerk Parameters [Movellan]/5(dxT)
  "xT, dxT, ddxT"/1 -> Demux1/1
  Demux1/3 -> Minimal Jerk Parameters [Movellan]/6(ddxT)
  Minimal Jerk Parameters [Movellan]/1(a) -> Enabled Subsystem/1(In1)
  Minus/1 -> Compare To Constant/1, Minus1/2, Minimal Jerk Parameters [Movellan]/7(T)
  Enabled Subsystem/1(Out1) -> Minimal Jerk/2(a [6x1])
  Compare To Constant/1 -> Switch/2, Enabled Subsystem/Enable
  Constant/1 -> Minus1/1
  Minus1/1 -> Switch/3
  Switch/1 -> Minimal Jerk/1(t)

== system nms3D_2021/Supraspinal Level/Subsystem/Swing Leg Control/Compute Acceleration Profiles with Minimal Jerk Approach/Minimal jerk Hip Pitch2 ==
  T_tot : Inport
  t_passed : Inport  Port=2
  "x0, dx0, ddx0" : Inport  Port=3
  "xT, dxT, ddxT" : Inport  Port=4
  Compare To Constant : simulink/Logic and Bit Operations/Compare To Constant  relop=>=  const=mParams.control.timelimit  OutDataTypeStr=boolean
  Constant : Constant  Value=mParams.control.timelimit
  Constant1 : Constant  Value=0
  Demux : Demux  Outputs=3
  Demux1 : Demux  Outputs=3
  Enabled Subsystem : Subsystem  TreatAsAtomicUnit=on
  Minimal Jerk : Subsystem
  Minimal Jerk Parameters [Movellan] : Subsystem
  Minus : Sum  Inputs=+-
  Minus1 : Sum  Inputs=+-
  Switch : Switch
  jerk : Outport
  wires:
  Minimal Jerk/1(j(t)) -> jerk/1
  T_tot/1 -> Minus/1
  t_passed/1 -> Minus/2
  Constant1/1 -> Switch/1
  Demux/1 -> Minimal Jerk Parameters [Movellan]/1(x0)
  Demux/2 -> Minimal Jerk Parameters [Movellan]/2(dx0)
  Demux/3 -> Minimal Jerk Parameters [Movellan]/3(ddx0)
  Demux1/1 -> Minimal Jerk Parameters [Movellan]/4(xT)
  "x0, dx0, ddx0"/1 -> Demux/1
  Demux1/2 -> Minimal Jerk Parameters [Movellan]/5(dxT)
  "xT, dxT, ddxT"/1 -> Demux1/1
  Demux1/3 -> Minimal Jerk Parameters [Movellan]/6(ddxT)
  Minimal Jerk Parameters [Movellan]/1(a) -> Enabled Subsystem/1(In1)
  Minus/1 -> Compare To Constant/1, Minus1/2, Minimal Jerk Parameters [Movellan]/7(T)
  Enabled Subsystem/1(Out1) -> Minimal Jerk/2(a [6x1])
  Compare To Constant/1 -> Switch/2, Enabled Subsystem/Enable
  Constant/1 -> Minus1/1
  Minus1/1 -> Switch/3
  Switch/1 -> Minimal Jerk/1(t)

== system nms3D_2021/Supraspinal Level/Subsystem/Swing Leg Control/Compute Acceleration Profiles with Minimal Jerk Approach/Minimal jerk Hip Pitch3 ==
  T_tot : Inport
  t_passed : Inport  Port=2
  "x0, dx0, ddx0" : Inport  Port=3
  "xT, dxT, ddxT" : Inport  Port=4
  Compare To Constant1 : simulink/Logic and Bit Operations/Compare To Constant  relop=>=  const=mParams.control.timelimit  OutDataTypeStr=boolean
  Constant : Constant  Value=mParams.control.timelimit
  Constant1 : Constant  Value=0
  Demux : Demux  Outputs=3
  Demux1 : Demux  Outputs=3
  Enabled Subsystem : Subsystem  TreatAsAtomicUnit=on
  Minimal Jerk : Subsystem
  Minimal Jerk Parameters [Movellan] : Subsystem
  Minus : Sum  Inputs=+-
  Minus1 : Sum  Inputs=+-
  Switch : Switch
  jerk : Outport
  wires:
  Minimal Jerk/1(j(t)) -> jerk/1
  T_tot/1 -> Minus/1
  t_passed/1 -> Minus/2
  Constant1/1 -> Switch/1
  Demux/1 -> Minimal Jerk Parameters [Movellan]/1(x0)
  Demux/2 -> Minimal Jerk Parameters [Movellan]/2(dx0)
  Demux/3 -> Minimal Jerk Parameters [Movellan]/3(ddx0)
  Demux1/1 -> Minimal Jerk Parameters [Movellan]/4(xT)
  "x0, dx0, ddx0"/1 -> Demux/1
  Demux1/2 -> Minimal Jerk Parameters [Movellan]/5(dxT)
  "xT, dxT, ddxT"/1 -> Demux1/1
  Demux1/3 -> Minimal Jerk Parameters [Movellan]/6(ddxT)
  Minimal Jerk Parameters [Movellan]/1(a) -> Enabled Subsystem/1(In1)
  Minus/1 -> Compare To Constant1/1, Minus1/2, Minimal Jerk Parameters [Movellan]/7(T)
  Enabled Subsystem/1(Out1) -> Minimal Jerk/2(a [6x1])
  Compare To Constant1/1 -> Switch/2, Enabled Subsystem/Enable
  Constant/1 -> Minus1/1
  Minus1/1 -> Switch/3
  Switch/1 -> Minimal Jerk/1(t)

== system nms3D_2021/Supraspinal Level/Subsystem/Swing Leg Control/Compute Acceleration Profiles with Minimal Jerk Approach/Minimal jerk Hip Roll4 ==
  T_tot : Inport
  t_passed : Inport  Port=2
  "x0, dx0, ddx0" : Inport  Port=3
  "xT, dxT, ddxT" : Inport  Port=4
  Constant1 : Constant  Value=0
  Demux : Demux  Outputs=3
  Demux1 : Demux  Outputs=3
  Minimal Jerk : Subsystem
  Minimal Jerk Parameters[Movellan] : Subsystem
  Minus : Sum  Inputs=+-
  Saturation : Saturate  UpperLimit=inf  LowerLimit=0.08
  jerk : Outport
  wires:
  Minimal Jerk/1(j(t)) -> jerk/1
  T_tot/1 -> Minus/1
  Minimal Jerk Parameters[Movellan]/1(a) -> Minimal Jerk/2(a [6x1])
  t_passed/1 -> Minus/2
  Constant1/1 -> Minimal Jerk/1(t)
  Minus/1 -> Saturation/1
  Demux/1 -> Minimal Jerk Parameters[Movellan]/1(x0)
  Demux/2 -> Minimal Jerk Parameters[Movellan]/2(dx0)
  Demux/3 -> Minimal Jerk Parameters[Movellan]/3(ddx0)
  Demux1/1 -> Minimal Jerk Parameters[Movellan]/4(xT)
  "x0, dx0, ddx0"/1 -> Demux/1
  Demux1/2 -> Minimal Jerk Parameters[Movellan]/5(dxT)
  "xT, dxT, ddxT"/1 -> Demux1/1
  Demux1/3 -> Minimal Jerk Parameters[Movellan]/6(ddxT)
  Saturation/1 -> Minimal Jerk Parameters[Movellan]/7(T)

== system nms3D_2021/Supraspinal Level/Subsystem/Swing Leg Control/Compute Target States/Balance Control lateral ==
  Left/Right : Inport
  Constant : Constant  Value=0
  Divide : Product  Inputs=**
  Divide1 : Product  Inputs=**
  Minus5 : Sum  Inputs=+++
  Minus6 : Sum  Inputs=+-
  Selector3 : Selector  InputPortWidth=3  IndexOptions=Index vector (dialog)  Indices=[3]  OutputSizes=1
  Selector4 : Selector  InputPortWidth=3  IndexOptions=Index vector (dialog)  Indices=[3]  OutputSizes=1
  Selector5 : Selector  InputPortWidth=3  IndexOptions=Index vector (dialog)  Indices=[3]  OutputSizes=1
  Switch : Switch  Criteria=u2 > Threshold
  theta_Hip_swing_target : Outport
  wires:
  Divide/1 -> Minus5/2
  [swh_lat] -> Minus5/1
  Switch/1 -> Minus6/2
  Divide1/1 -> Minus5/3
  [AnklePosR_rot] -> Selector3/1
  Minus6/1 -> Divide1/1
  Left/Right/1 -> Switch/2
  [AnklePosL_rot] -> Selector4/1
  [cv_lat] -> Divide/2
  [cd_lat] -> Divide1/2
  Selector4/1 -> Switch/1
  Selector3/1 -> Switch/3
  [CoM_Velocity_rot] -> Selector5/1
  Selector5/1 -> Divide/1
  Constant/1 -> Minus6/1
  Minus5/1 -> theta_Hip_swing_target/1

== system nms3D_2021/Supraspinal Level/Subsystem/Swing Leg Control/Compute Target States/Balance Control saggital ==
  Left/Right : Inport
  Early Late : Inport  Port=2
  Constant : Constant  Value=0
  Constant1 : Constant  Commented=on  Value=1.5
  Constant2 : Constant  Value=ICs.trunk.vx0
  Divide{,1..3} (4 alike) : Product  Inputs=**
  Enabled Subsystem : Subsystem  TreatAsAtomicUnit=on
  From2 : From  Commented=on  GotoTag=ca  TagVisibility=global
  Minus : Sum  Inputs=+-
  Minus5 : Sum  Inputs=+++++
  Minus6 : Sum  Inputs=+-
  Product : Product  Commented=on
  Scope : Scope
  Selector3 : Selector  InputPortWidth=3  IndexOptions=Index vector (dialog)  Indices=[1]  OutputSizes=1
  Selector4 : Selector  InputPortWidth=3  IndexOptions=Index vector (dialog)  Indices=[1]  OutputSizes=1
  Selector5 : Selector  InputPortWidth=3  IndexOptions=Index vector (dialog)  Indices=[1]  OutputSizes=1
  Switch : Switch  Criteria=u2 > Threshold
  theta_Hip_swing_target : Outport
  tag scope: d=global, v_mid=global
  wires:
  [swh] -> Minus5/1
  Switch/1 -> Minus6/2
  [AnklePosR_rot] -> Selector4/1
  Minus6/1 -> Divide1/1, [d]
  Left/Right/1 -> Switch/2
  [AnklePosL_rot] -> Selector3/1
  [cv] -> Divide/2
  [cd] -> Divide1/2
  Selector3/1 -> Switch/1
  Selector4/1 -> Switch/3
  Divide/1 -> Minus5/2
  [CoM_Velocity_rot] -> Selector5/1
  Constant/1 -> Minus6/1
  Divide1/1 -> Minus5/3
  Minus5/1 -> theta_Hip_swing_target/1
  Selector5/1 -> Enabled Subsystem/1(CoM Vel), Divide/1
  Early Late/1 -> Enabled Subsystem/Trigger
  Enabled Subsystem/1(CoM Vel at Midswing) -> Minus/2, Scope/1, [v_mid]
  From2/1 -> Product/1
  Constant2/1 -> Divide3/1, Minus/1
  [c4] -> Divide2/1
  Minus/1 -> Divide2/2
  Divide2/1 -> Minus5/5
  [c3] -> Divide3/2
  Divide3/1 -> Minus5/4

== system nms3D_2021/Supraspinal Level/Subsystem/Swing Leg Control/Inverse Dynamics: Left Leg/Inverse Dynamics ==
  note: Augment Joint Vectors: In order to compute appropriate gravitational and velocity dependend forces, the joint angle and joint angle acceleration vectors are augmented by the position and velocity of the body in space.
  Joint Angles [rad] : Inport
  Joint Angle Velocities [rad/s] : Inport  Port=2
  Joint  Acceleration [rad/s^2] : Inport  Port=3
  Rotation Trunk [rad] : Inport  Port=4
  Trunk Position [m] : Inport  Port=5
  Rotation Velocity Trunk [rad/s] : Inport  Port=6
  Trunk Velocity [m/s] : Inport  Port=7
  Desired Acceleration [rad/s^2] : Inport  Port=8
  Enable : EnablePort  ZeroCross=off
  Constant : Constant  Value=zeros(6,1)
  Inverse Dynamics : Subsystem
  Inverse Dynamics1 : Subsystem  Commented=on
  Mux : Mux  Inputs=3
  Mux1 : Mux  Inputs=3
  Mux2 : Mux  Inputs=2
  Mux4 : Mux  Inputs=2
  " Desired Torques" : Outport  VectorParamsAs1DForOutWhenUnconnected=off
  Interaction Wrench : Outport  Port=2  VectorParamsAs1DForOutWhenUnconnected=off
  wires:
  Trunk Position [m]/1 -> Mux1/1
  Inverse Dynamics/1(Desired Torques) -> " Desired Torques"/1
  Mux1/1 -> Inverse Dynamics/1(Config)
  Rotation Trunk [rad]/1 -> Mux1/2
  Mux/1 -> Inverse Dynamics/2(JointVel)
  Mux2/1 -> Inverse Dynamics/3(Des. JointAccel)
  Inverse Dynamics/2(Interaction Wrench Left) -> Interaction Wrench/1
  Constant/1 -> Mux4/1, Mux2/1
  Mux4/1 -> Inverse Dynamics/4(Real JointAccel)
  Trunk Velocity [m/s]/1 -> Mux/1
  Rotation Velocity Trunk [rad/s]/1 -> Mux/2
  Joint Angles [rad]/1 -> Mux1/3
  Joint Angle Velocities [rad/s]/1 -> Mux/3
  Joint  Acceleration [rad/s^2]/1 -> Mux4/2
  Desired Acceleration [rad/s^2]/1 -> Mux2/2

== system nms3D_2021/Supraspinal Level/Subsystem/Swing Leg Control/Inverse Dynamics: Left Leg/Sensor Data from Body Layer ==
  Constant : Constant  Commented=on  Value=0
  Constant1 : Constant  Value=zeros(3,1)
  From3 : From  Commented=on  GotoTag=TrunkRot_lat  TagVisibility=global
  From4 : From  Commented=on  GotoTag=TrunkRot_sag  TagVisibility=global
  From44 : From  Commented=on  GotoTag=RotationalVelocityTrunk  TagVisibility=global
  From46 : From  Commented=on  GotoTag=TranslationalVelocityTrunk  TagVisibility=global
  Gain : Gain  Gain=0
  Gain1 : Gain  Gain=0
  Mux : Mux  Commented=on  Inputs=3
  Sensor Delay 1 : eeGeneralControl/Low-Pass Filter (Discrete or Continuous)  K=1  T=0.01  B=inf  A=-inf  init_option=Inherited from block input  x0=0  Ts=0
  Sensor Delay 2 : eeGeneralControl/Low-Pass Filter (Discrete or Continuous)  K=1  T=0.01  B=inf  A=-inf  init_option=Inherited from block input  x0=0  Ts=0
  Sensor Delay 3 : eeGeneralControl/Low-Pass Filter (Discrete or Continuous)  K=1  T=0.01  B=inf  A=-inf  init_option=Inherited from block input  x0=0  Ts=0
  Joint Angles [rad] : Outport
  Joint Angle Velocities [rad/s] : Outport  Port=2
  Joint Angle Accelerations [rad/s^2] : Outport  Port=3
  " Rotation Trunk [rad]" : Outport  Port=4
  Trunk Position [m] : Outport  Port=5
  Rotation Velocity Trunk [rad/s] : Outport  Port=6
  Trunk Velocity [m/s] : Outport  Port=7
  wires:
  [Llegq] -> Sensor Delay 3/1
  [Llegdq] -> Sensor Delay 1/1
  Sensor Delay 3/1 -> Joint Angles [rad]/1
  Sensor Delay 1/1 -> Joint Angle Velocities [rad/s]/1
  [CoM_Position] -> Trunk Position [m]/1
  [Llegddq] -> Sensor Delay 2/1
  Sensor Delay 2/1 -> Joint Angle Accelerations [rad/s^2]/1
  From3/1 -> Mux/1
  Constant/1 -> Mux/2
  From4/1 -> Mux/3
  [RotationTrunk] -> " Rotation Trunk [rad]"/1
  Gain/1 -> Rotation Velocity Trunk [rad/s]/1
  Gain1/1 -> Trunk Velocity [m/s]/1
  Constant1/1 -> Gain1/1, Gain/1

== system nms3D_2021/Supraspinal Level/Subsystem/Swing Leg Control/Inverse Dynamics: Right Leg/Inverse Dynamics1 ==
  note: Augment Joint Vectors: In order to compute appropriate gravitational and velocity dependend forces, the joint angle and joint angle acceleration vectors are augmented by the position and velocity of the body in space.
  Joint Angles [rad] : Inport
  Joint Angle Velocities [rad/s] : Inport  Port=2
  Joint  Acceleration [rad/s^2] : Inport  Port=3
  Rotation Trunk [rad] : Inport  Port=4
  Trunk Position [m] : Inport  Port=5
  Rotation Velocity Trunk [rad/s] : Inport  Port=6
  Trunk Velocity [m/s] : Inport  Port=7
  Desired Acceleration [rad/s^2] : Inport  Port=8
  Enable : EnablePort  ZeroCross=off
  Constant : Constant  Value=zeros(6,1)
  Inverse Dynamics : Subsystem
  Mux : Mux  Inputs=3
  Mux1 : Mux  Inputs=3
  Mux2 : Mux  Inputs=2
  Mux4 : Mux  Inputs=2
  " Desired Torques" : Outport  VectorParamsAs1DForOutWhenUnconnected=off
  Interaction Wrench : Outport  Port=2  VectorParamsAs1DForOutWhenUnconnected=off
  wires:
  Trunk Position [m]/1 -> Mux1/1
  Inverse Dynamics/1(Desired Torques) -> " Desired Torques"/1
  Mux1/1 -> Inverse Dynamics/1(Config)
  Rotation Trunk [rad]/1 -> Mux1/2
  Mux/1 -> Inverse Dynamics/2(JointVel)
  Mux2/1 -> Inverse Dynamics/3(Des. JointAccel)
  Mux4/1 -> Inverse Dynamics/4(Real JointAccel)
  Inverse Dynamics/2(Interaction Wrench Left) -> Interaction Wrench/1
  Trunk Velocity [m/s]/1 -> Mux/1
  Rotation Velocity Trunk [rad/s]/1 -> Mux/2
  Joint Angles [rad]/1 -> Mux1/3
  Joint Angle Velocities [rad/s]/1 -> Mux/3
  Constant/1 -> Mux4/1, Mux2/1
  Joint  Acceleration [rad/s^2]/1 -> Mux4/2
  Desired Acceleration [rad/s^2]/1 -> Mux2/2

== system nms3D_2021/Supraspinal Level/Subsystem/Swing Leg Control/Inverse Dynamics: Right Leg/Sensor Data from Body Layer1 ==
  Constant1 : Constant  Value=zeros(3,1)
  From44 : From  Commented=on  GotoTag=RotationalVelocityTrunk  TagVisibility=global
  From46 : From  Commented=on  GotoTag=TranslationalVelocityTrunk  TagVisibility=global
  Gain : Gain  Gain=0
  Gain1 : Gain  Gain=0
  Sensor Delay 1 : eeGeneralControl/Low-Pass Filter (Discrete or Continuous)  K=1  T=0.01  B=inf  A=-inf  init_option=Inherited from block input  x0=0  Ts=0
  Sensor Delay 2 : eeGeneralControl/Low-Pass Filter (Discrete or Continuous)  K=1  T=0.01  B=inf  A=-inf  init_option=Inherited from block input  x0=0  Ts=0
  Sensor Delay 3 : eeGeneralControl/Low-Pass Filter (Discrete or Continuous)  K=1  T=0.01  B=inf  A=-inf  init_option=Inherited from block input  x0=0  Ts=0
  Joint Angles [rad] : Outport
  Joint Angle Velocities [rad/s] : Outport  Port=2
  Joint Angle Accelerations [rad/s^2] : Outport  Port=3
  " Rotation Trunk [rad]" : Outport  Port=4
  Trunk Position [m] : Outport  Port=5
  Rotation Velocity Trunk [rad/s] : Outport  Port=6
  Trunk Velocity [m/s] : Outport  Port=7
  wires:
  [Rlegq] -> Sensor Delay 3/1
  [Rlegdq] -> Sensor Delay 1/1
  Sensor Delay 3/1 -> Joint Angles [rad]/1
  Sensor Delay 1/1 -> Joint Angle Velocities [rad/s]/1
  [CoM_Position] -> Trunk Position [m]/1
  [Rlegddq5] -> Sensor Delay 2/1
  Sensor Delay 2/1 -> Joint Angle Accelerations [rad/s^2]/1
  [RotationTrunk] -> " Rotation Trunk [rad]"/1
  Gain/1 -> Rotation Velocity Trunk [rad/s]/1
  Gain1/1 -> Trunk Velocity [m/s]/1
  Constant1/1 -> Gain1/1, Gain/1
